simulink model "luinverse_tut"  (Simulink 4.00)
settings: Solver=FixedStepDiscrete  StartTime=0.0  StopTime=10.0  RelTol=1e-3
PostLoadFcn:
  | set_param(gcs,'SimulationCommand','Update')
libraries: dspinverses x1, dspsrcs3 x1, dspmtrx3 x1
settings Model: RequirementInfo=9  LastModifiedBy=dfass  LimitDataPoints=off  ExtModeTrigMode=oneshot  ExtModeArmWhenConnect=off  BlockReductionOpt=off

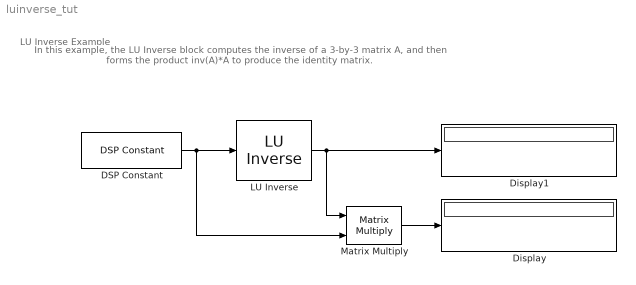
== system luinverse_tut ==
  note: LU Inverse Example
  note: In this example, the LU Inverse block computes the inverse of a 3-by-3 matrix A,
      | and then forms the product inv(A)*A to produce the identity matrix.
  " LU Inverse" : dspinverses/ LU Inverse
  DSP Constant : dspsrcs3/DSP Constant  Value=[1 -2 3;4 0 6;2 -1 3]  InterpretAs1D=off  SampleMode=Discrete  Ts=1  FramebasedOutput=off
  Display : Display
      settings: Format=short
  Display1 : Display
      settings: Format=short
  Matrix Multiply : dspmtrx3/Matrix Multiply  numInputPorts=2  OptimizationLevel=None
  wires:
  DSP Constant/1 -> " LU Inverse"/1, Matrix Multiply/2
  " LU Inverse"/1 -> Display1/1, Matrix Multiply/1
  Matrix Multiply/1 -> Display/1
